simulink model "battery_status"  (R2020b)
settings: Solver=VariableStepAuto  StartTime=0.0  StopTime=10.0  RelTol=1e-3
undefined symbols (not defined in the file): batteryHV, DiscIntNeverNeededParam, hvBatterySOC_pct, nominalCapacity_kWh
settings Model: DataDictionary=battery_status.sldd  Creator=Dmitry  LastModifiedBy=Dmitry

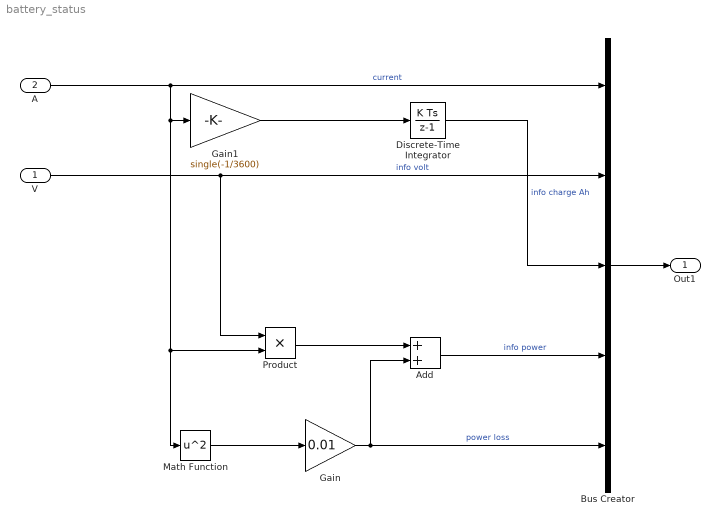
== system battery_status ==
  V : Inport
  A : Inport  Port=2
  Add : Sum
  Bus Creator : BusCreator  Inputs=5  OutDataTypeStr=Bus: Bus
  Discrete-Time Integrator : DiscreteIntegrator  gainval=nominalCapacity_kWh/batteryHV.packVoltage_V*1000*hvBatterySOC_pct/100  InitialCondition=8  SampleTime=-1  OutDataTypeStr=single  ICPrevOutput=DiscIntNeverNeededParam  ICPrevScaledInput=DiscIntNeverNeededParam
  Gain : Gain  Gain=0.01
  Gain1 : Gain  Gain=single(-1/3600)
  Math Function : Math  Operator=square  SaturateOnIntegerOverflow=on
  Product : Product
  Out1 : Outport  OutDataTypeStr=Bus: Bus
  wires:
  Add/1 -> Bus Creator/4  "info power"
  A/1 -> Math Function/1, Product/2, Gain1/1, Bus Creator/1  "current"
  Math Function/1 -> Gain/1
  Gain/1 -> Add/2, Bus Creator/5  "power loss"
  Product/1 -> Add/1
  Gain1/1 -> Discrete-Time Integrator/1
  Discrete-Time Integrator/1 -> Bus Creator/3  "info charge Ah"
  Bus Creator/1 -> Out1/1
  V/1 -> Bus Creator/2, Product/1  "info volt"
